simulink model "Grid_SensorLayout_SpatialAllignment_Clustering"  (R2018a)
settings: Solver=FixedStepAuto  StartTime=0.0  StopTime=SimulationTime  FixedStep=SamplingTime  RelTol=1e-3
values from neighbouring files (symbols this model uses):
  ValidateGRID = true    [SensorFusion_Script0_main.m]
  ValidateLAYOUT = true    [SensorFusion_Script0_main.m]
  VisualizeCLUSTERING = true    [SensorFusion_Script0_main.m]
undefined symbols (not defined in the file or in its folder): ACTIVATE_CAM, ACTIVATE_RAD, CAM1_detTimeStamp, CAM1_MeasNoise, CAM1_objClassID, CAM1_PX, CAM1_PY, CAM1_VX, CAM1_VY, CAM2_detTimeStamp, CAM2_MeasNoise, CAM2_objClassID, CAM2_PX, CAM2_PY, CAM2_VX, CAM2_VY, CAM3_detTimeStamp, CAM3_MeasNoise, CAM3_objClassID, CAM3_PX, CAM3_PY, CAM3_VX, CAM3_VY, CAM4_detTimeStamp, CAM4_MeasNoise, CAM4_objClassID, CAM4_PX, CAM4_PY, CAM4_VX, CAM4_VY, CAM5_detTimeStamp, CAM5_MeasNoise, CAM5_objClassID, CAM5_PX, CAM5_PY, CAM5_VX, CAM5_VY, CAM6_detTimeStamp, CAM6_MeasNoise, CAM6_objClassID, CAM6_PX, CAM6_PY, CAM6_VX, CAM6_VY, CAM7_detTimeStamp, CAM7_MeasNoise, CAM7_objClassID, CAM7_PX, CAM7_PY, CAM7_VX, CAM7_VY, CAM8_detTimeStamp, CAM8_MeasNoise, CAM8_objClassID, CAM8_PX, CAM8_PY, CAM8_VX, CAM8_VY, CAM_nMeas, CAM_TYPE ... (+171)
libraries: simulink_extras x4
(part 10 of 10)

== matlab function Grid_SensorLayout_SpatialAllignment_Clustering/Radar_and_Camera_cluster_plots/VISUALIZE_CLUSTERING/MATLAB Function ==
  data: RadCluster input; RadMeas input; CamMeas input; CamCluster input
function vizClusters(RadCluster, RadMeas, CamMeas, CamCluster)
  
     nPts = 100;
     px_Meas = single(zeros(1,100)); 
     py_Meas = single(zeros(1,100));
     Cos_Sin_theta = single(zeros(2,nPts));
     mu = single(zeros(2,nPts));
     ThetaMax = single(2*pi); ThetaMin = single(0);
     dTheta = (ThetaMax - ThetaMin)/(nPts - 1);
     Theta = ThetaMin:dTheta:ThetaMax;
     Cos_Sin_theta(1,:) = cos(Theta);
     Cos_Sin_theta(2,:) = sin(Theta);
     level = sqrt(5); 
     sigma = sqrt(5);
     
     figure(2);
     subplot(2,1,1);
     for i = 1:RadCluster.nClusters  % plot Cluster
         px = RadCluster.ClusterCenter(1,i);
         py = RadCluster.ClusterCenter(2,i);
         %Sigma_sqrt = sqrtm(RadCluster.ClusterCovariance(:,:,i));
         Sigma_sqrt = single([sigma,0;0,sigma]);
         val = level.*(Sigma_sqrt*Cos_Sin_theta);
         mu(1,:) = repmat(px, 1, nPts);
         mu(2,:) = repmat(py, 1, nPts);
         xy = mu + val;
         plot(px, py, 'x','markersize',8, 'color', 'k');hold on;
         plot(xy(1,:), xy(2,:), '-', 'LineWidth',1, 'color', 'r');hold on;
     end
     nRadarMeas = RadMeas.ValidCumulativeMeasCount(end);
     for i = 1:nRadarMeas  % plot radar measurements
         px_Meas(1,i) = RadMeas.MeasArray(1,i);
         py_Meas(1,i) = RadMeas.MeasArray(2,i);
     end
     plot(px_Meas(1,1:nRadarMeas), py_Meas(1,1:nRadarMeas), '.', 'markersize',5, 'color', 'r');hold on;
     axis equal;  grid on; hold off;
     xlabel('x(m)');ylabel('y(m)');
     title('DBSCAN Clustering of Radar Measurements', 'FontSize', 10);
     set(gca,'XLim',[-120 120])
     set(gca,'YLim',[-40 40])
     
     subplot(2,1,2);
     for i = 1:CamCluster.nClusters
         px = CamCluster.ClusterCenter(1,i);
         py = CamCluster.ClusterCenter(2,i);
         %Sigma_sqrt = sqrtm(CamCluster.ClusterCovariance(:,:,i));
         Sigma_sqrt = single([sigma,0;0,sigma]);
         val = level.*(Sigma_sqrt*Cos_Sin_theta);
         mu(1,:) = repmat(px, 1, nPts);
         mu(2,:) = repmat(py, 1, nPts);
         xy = mu + val;
         plot(px, py, 'x','markersize',8, 'color', 'k');hold on;
         plot(xy(1,:), xy(2,:), '-', 'LineWidth',1, 'color', 'b');hold on;
     end
     nCameraMeas = CamMeas.ValidCumulativeMeasCount(end);
     for i = 1:nCameraMeas  % plot radar measurements
         px_Meas(1,i) = CamMeas.MeasArray(1,i);
         py_Meas(1,i) = CamMeas.MeasArray(2,i);
     end
     plot(px_Meas(1,1:nCameraMeas), py_Meas(1,1:nCameraMeas), '.', 'markersize',5, 'color', 'b');hold on;
     axis equal;  grid on; hold off;
     xlabel('x(m)');ylabel('y(m)');
     title('NN Clustering of Camera Measurements', 'FontSize', 10);
     set(gca,'XLim',[-120 120])
     set(gca,'YLim',[-40 40])
end

== matlab function Grid_SensorLayout_SpatialAllignment_Clustering/OBJECT_TRACKER_SENSOR_FUSION/SENSOR_LAYOUT_AND_CHRACTERIZATION/ValidateSensorLayout/MATLAB Function ==
  data: RadarParam input; CameraParam input
function RadarSensors(RadarParam,  CameraParam)


         % RADARS =========================================================
         nSensorTypesRAD = length(RadarParam.RadarIntrinsics);
         nSensorsRAD = length(RadarParam.RadarExtrinsics);
         SensorINTRINSICparam = RadarParam.RadarIntrinsics;
         nPts = 100; DEG2RAD = pi/180;
         SensorFOVPtsCartesian = struct;
         SensorFOVPtsCartesian.SensorID = uint16(0);
         SensorFOVPtsCartesian.XCoord = single(zeros(1,nPts + 2));
         SensorFOVPtsCartesian.YCoord = single(zeros(1,nPts + 2));
         SensorFOVPtsCartesian = SensorFOVPtsCartesian(ones(1, nSensorTypesRAD));
         
         % Set the Radar intrinsics
         for idx = 1:nSensorTypesRAD
             %FOVPts = GenerateFOVBoundaryPointsCartesian(SensorINTRINSICparam(idx).MaxRange, SensorINTRINSICparam(idx).MaxAzimuth, nPts);
             FOVMaxAzimuth = SensorINTRINSICparam(idx).MaxAzimuth;
             FOVMaxRange = SensorINTRINSICparam(idx).MaxRange;
             FOV_boundary = single(zeros(2,nPts + 2));
             dTheta = 2*FOVMaxAzimuth/(nPts-1);
             thetaInit = -FOVMaxAzimuth;
             FOV_boundary(1,1) = single(0);
             FOV_boundary(2,1) = single(0);
             for i = 1:nPts
                 theta = thetaInit + (i -1)*dTheta;
                 FOV_boundary(1,i) = FOVMaxRange*cos(theta*DEG2RAD);
                 FOV_boundary(2,i) = FOVMaxRange*sin(theta*DEG2RAD);
             end
             FOV_boundary(:,end) = FOV_boundary(:,1);
             %FOV_boundary(:,end) = single(zeros(size(FOV_boundary(:,1))));
             SensorFOVPtsCartesian(idx).XCoord = FOV_boundary(1,:);
             SensorFOVPtsCartesian(idx).YCoord = FOV_boundary(2,:);
             SensorFOVPtsCartesian(idx).SensorID = uint16(idx);
         end
         
         % Set Radar Extrinsics
         FOVPtsEGOframeRAD = struct;
         FOVPtsEGOframeRAD.Xcoord = single(zeros(1,nPts + 2));
         FOVPtsEGOframeRAD.Ycoord = single(zeros(1,nPts + 2));
         FOVPtsEGOframeRAD = FOVPtsEGOframeRAD(ones(1, nSensorsRAD));
         PtsLocalFrame = single(zeros(2,nPts + 2));
         for idx = 1:nSensorsRAD
             snsrType = RadarParam.RadarExtrinsics(idx).RadarType;
             PtsLocalFrame(1,:) = SensorFOVPtsCartesian(snsrType).XCoord(1,:);
             PtsLocalFrame(2,:) = SensorFOVPtsCartesian(snsrType).YCoord(1,:);
             RotMatrix = RadarParam.RadarExtrinsics(idx).RotMat2D; 
             TranslationVector = RadarParam.RadarExtrinsics(idx).TranslationVec;
             TranslationVector = repmat(TranslationVector, 1, nPts + 2);
             PtsEGOframe = RotMatrix * PtsLocalFrame + TranslationVector;
             FOVPtsEGOframeRAD(idx).Xcoord = PtsEGOframe(1,:);
             FOVPtsEGOframeRAD(idx).Ycoord = PtsEGOframe(2,:);
         end
         
         % CAMERAS =========================================================
         nSensorTypesCAM = length(CameraParam.CameraIntrinsics);
         nSensorsCAM = length(CameraParam.CameraExtrinsics);
         SensorINTRINSICparam = CameraParam.CameraIntrinsics;
         nPts = 100; DEG2RAD = pi/180;
         SensorFOVPtsCartesian = struct;
         SensorFOVPtsCartesian.SensorID = uint16(0);
         SensorFOVPtsCartesian.XCoord = single(zeros(1,nPts + 2));
         SensorFOVPtsCartesian.YCoord = single(zeros(1,nPts + 2));
         SensorFOVPtsCartesian = SensorFOVPtsCartesian(ones(1, nSensorTypesCAM));
         
         % Set the Camera intrinsics
         for idx = 1:nSensorTypesCAM
             %FOVPts = GenerateFOVBoundaryPointsCartesian(SensorINTRINSICparam(idx).MaxRange, SensorINTRINSICparam(idx).MaxAzimuth, nPts);
             FOVMaxAzimuth = SensorINTRINSICparam(idx).MaxAzimuth;
             FOVMaxRange = SensorINTRINSICparam(idx).MaxRange;
             FOV_boundary = single(zeros(2,nPts + 2));
             dTheta = 2*FOVMaxAzimuth/(nPts-1);
             thetaInit = -FOVMaxAzimuth;
             FOV_boundary(1,1) = single(0);
             FOV_boundary(2,1) = single(0);
             for i = 1:nPts
                 theta = thetaInit + (i -1)*dTheta;
                 FOV_boundary(1,i) = FOVMaxRange*cos(theta*DEG2RAD);
                 FOV_boundary(2,i) = FOVMaxRange*sin(theta*DEG2RAD);
             end
             FOV_boundary(:,end) = FOV_boundary(:,1);
             %FOV_boundary(:,end) = single(zeros(size(FOV_boundary(:,1))));
             SensorFOVPtsCartesian(idx).XCoord = FOV_boundary(1,:);
             SensorFOVPtsCartesian(idx).YCoord = FOV_boundary(2,:);
             SensorFOVPtsCartesian(idx).SensorID = uint16(idx);
         end
         
         % Set Camera Extrinsics
         FOVPtsEGOframeCAM = struct;
         FOVPtsEGOframeCAM.Xcoord = single(zeros(1,nPts + 2));
         FOVPtsEGOframeCAM.Ycoord = single(zeros(1,nPts + 2));
         FOVPtsEGOframeCAM = FOVPtsEGOframeCAM(ones(1, nSensorsCAM));
         PtsLocalFrame = single(zeros(2,nPts + 2));
         for idx = 1:nSensorsCAM
             snsrType = CameraParam.CameraExtrinsics(idx).CameraType;
             PtsLocalFrame(1,:) = SensorFOVPtsCartesian(snsrType).XCoord(1,:);
             PtsLocalFrame(2,:) = SensorFOVPtsCartesian(snsrType).YCoord(1,:);
             RotMatrix = CameraParam.CameraExtrinsics(idx).RotMat2D; 
             TranslationVector = CameraParam.CameraExtrinsics(idx).TranslationVec;
             TranslationVector = repmat(TranslationVector, 1, nPts + 2);
             PtsEGOframe = RotMatrix * PtsLocalFrame + TranslationVector;
             FOVPtsEGOframeCAM(idx).Xcoord = PtsEGOframe(1,:);
             FOVPtsEGOframeCAM(idx).Ycoord = PtsEGOframe(2,:);
         end
         
         
         
         % Plot The Radar Layout
         figure(1); fontSize = 10;
         subplot(2,2,1);
         title('Radar Layout')
         VehDim = [3.7, 3.7, -1, -1,3.7; 0.9, -0.9, -0.9, 0.9,0.9];
         plot(VehDim(1,:), VehDim(2,:),'-','color','k','linewidth',5); hold on;
         for i = 1:nSensorsRAD
             plot(FOVPtsEGOframeRAD(i).Xcoord, FOVPtsEGOframeRAD(i).Ycoord,'-','linewidth',1); hold on;
         end
         title('Radar Layout', 'FontSize', fontSize);
         axis equal; grid on;hold off;
         xlabel('x coordinate (m)'); ylabel('y coordinate (m)');
         set(gca,'XLim',[-160 210]); set(gca,'YLim',[-110 110]); 
         
         
         % Plot The Camera Layout
         subplot(2,2,2);
         VehDim = [3.7, 3.7, -1, -1,3.7; 0.9, -0.9, -0.9, 0.9,0.9];
         plot(VehDim(1,:), VehDim(2,:),'-','color','k','linewidth',5); hold on;
         for i = 1:nSensorsCAM
             plot(FOVPtsEGOframeCAM(i).Xcoord, FOVPtsEGOframeCAM(i).Ycoord,'-','linewidth',1); hold on;
         end
         title('Camera Layout', 'FontSize', fontSize);
         axis equal; grid on;hold off;
         xlabel('x coordinate (m)'); ylabel('y coordinate (m)');
         set(gca,'XLim',[-160 210]); set(gca,'YLim',[-110 110]); 
         
         
         % Plot The Radar and Camera Layout
         subplot(2,2,3);
         VehDim = [3.7, 3.7, -1, -1,3.7; 0.9, -0.9, -0.9, 0.9,0.9];
         plot(VehDim(1,:), VehDim(2,:),'-','color','k','linewidth',5); hold on;
         for i = 1:nSensorsRAD
             plot(FOVPtsEGOframeRAD(i).Xcoord, FOVPtsEGOframeRAD(i).Ycoord,'-','linewidth',1); hold on;
         end
         for i = 1:nSensorsCAM
             plot(FOVPtsEGOframeCAM(i).Xcoord, FOVPtsEGOframeCAM(i).Ycoord,'-','linewidth',1); hold on;
         end
         title('Radar + Camera Layout', 'FontSize', fontSize);
         axis equal; grid on;hold off;
         xlabel('x coordinate (m)'); ylabel('y coordinate (m)');
         set(gca,'XLim',[-160 210]); set(gca,'YLim',[-110 110]); 
         
         hold off;
end

== matlab function Grid_SensorLayout_SpatialAllignment_Clustering/Radar_and_Camera_cluster_plots/SEGREGATE_CLUSTER/MATLAB Function ==
  data: SENSORMeasCTS input; MeasArray output; SENSOR_CLUSTERS input; MeasCovariance output; ClusterRef output; ValidMeasCount output; ValidCumulativeMeasCount output
function [MeasArray, MeasCovariance, ClusterRef, ValidMeasCount, ValidCumulativeMeasCount] = SEGREGATE_CLUSTER(SENSORMeasCTS, SENSOR_CLUSTERS)
     
    nSensors = length(SENSORMeasCTS.ValidCumulativeMeasCount); % total number of sensors installed around the ego vehicle
    nMeas = SENSORMeasCTS.ValidCumulativeMeasCount(end);       % total number of measurements received  
    nSnsrClsters = SENSOR_CLUSTERS.nClusters;                  % total number of measurement clusters (all radars combined)
    countTotal = int16(0);
            
    % Initializations for the output
    MeasArray = single(zeros(2 , 1200));
    MeasCovariance = single(zeros(2, 2, 1200));
    ClusterRef = uint16(zeros(2 , 1200));
    ValidMeasCount = uint16(zeros(1,6));
    x = single(zeros(2,1)); R = single(zeros(2,2)); xSpread = single(zeros(2,2));
            
    for snsrIdx = 1:nSensors            % iterate over each of the sensors
        for idxClstr = 1:nSnsrClsters   % for each of the Radar clusters
            % 1. extract the associated cluster IDs
            clusterID = uint16(idxClstr); 
            % 2. extract the measurement IDs forming the cluster
            measIDsIndex = find(clusterID == SENSOR_CLUSTERS.ClusterToMeasAssignment(1,1:nMeas)); 
            % 3. extract the associated measurement IDs for each of the sensors
            measIDs = measIDsIndex(snsrIdx == SENSORMeasCTS.MeasRef(2,measIDsIndex)); 
            if(~isempty(measIDs))
               countTotal = countTotal + 1;
               weight = 1/length(measIDs);
               x(:) = 0; R(:) = 0;xSpread(:) = 0;
               for idxMeas = 1:length(measIDs)   % for each of the extracted measurements compute the weighted mean and covariance
                   x = x + weight.*SENSORMeasCTS.MeasArray(:,measIDs(idxMeas));
                   R = R + weight.*SENSORMeasCTS.MeasCovariance(:,:,measIDs(idxMeas));
               end
               for idxMeas = 1:length(measIDs)   % compute the spread of the mean
                   z = SENSORMeasCTS.MeasArray(:,measIDs(idxMeas));
                   xSpread = xSpread + weight.*( (x - z)*(x - z)' );
               end
               %R = R + xSpread;
               MeasArray(:,countTotal) = x;
               MeasCovariance(:,:,countTotal) = R;
               ClusterRef(1,countTotal) = snsrIdx;
               ClusterRef(2,countTotal) = clusterID;
               ValidMeasCount(1,snsrIdx) = ValidMeasCount(1,snsrIdx) + 1;
            end
        end
    end
    ValidCumulativeMeasCount = cumsum(ValidMeasCount);
end
